simulink model "Nominal_CBF_ACC"  (R2018a)
settings: Solver=FixedStepAuto  StartTime=0.0  StopTime=Tsim  FixedStep=0.001  RelTol=1e-3
InitFcn:
  | tic;
  | disp('Simulation started...');
StopFcn:
  | elapsedTime_nominal = toc; % Stop timer when simulation ends
  | fprintf('Simulation Time: %.6f seconds\n', elapsedTime_nominal);
  | 
  | % out_nominal = out;
undefined symbols (not defined in the file): case_num, D0, epsilon, f0, f1, f2, g, gamma, k, k_fric, m, magnitude, omega0, p_omega, psc, v0, vd, x10, x20
settings Model: Creator=Administrator  LastModifiedBy=hieunguyen412
settings DataIOCC: ReturnWorkspaceOutputs=on
settings SFSimCC: SimUseLocalCustomCode=on
settings RTWCC: RTWUseLocalCustomCode=on

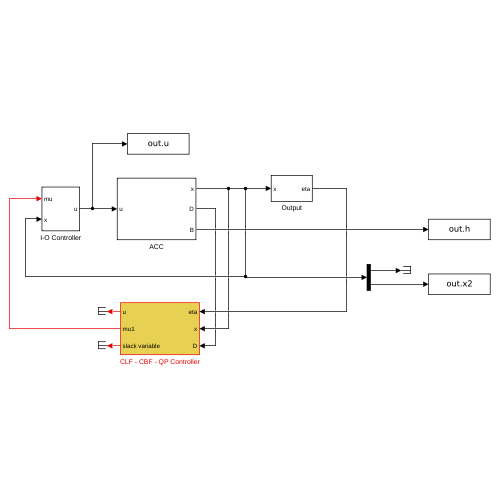
[thumbnail: Simulink's stored preview of the top-level diagram]
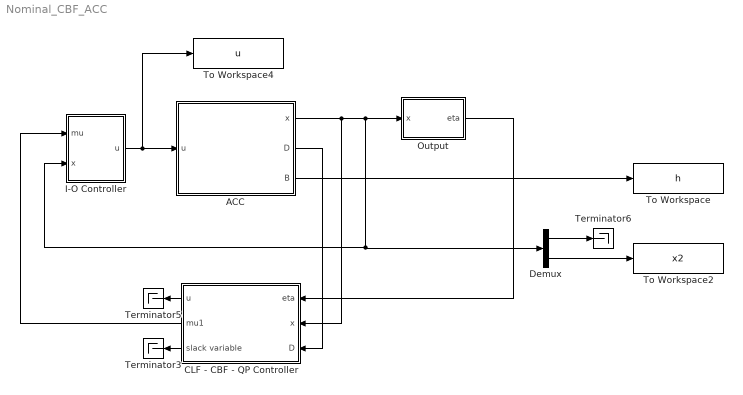
== system Nominal_CBF_ACC ==
  ACC : Subsystem
  CLF - CBF - QP Controller : Subsystem
  Demux : Demux  Outputs=2
  I-O Controller : Subsystem
  Output : Subsystem
  Terminator3 : Terminator
  Terminator5 : Terminator
  Terminator6 : Terminator
  To Workspace : ToWorkspace  VariableName=h  SampleTime=-1
  To Workspace2 : ToWorkspace  VariableName=x2  SampleTime=-1
  To Workspace4 : ToWorkspace  VariableName=u  SampleTime=-1
  wires:
  ACC/1(x) -> CLF - CBF - QP Controller/2(x), I-O Controller/2(x), Demux/1, Output/1(x)
  I-O Controller/1(u) -> To Workspace4/1, ACC/1(u)
  CLF - CBF - QP Controller/3(slack variable) -> Terminator3/1
  CLF - CBF - QP Controller/1(u) -> Terminator5/1
  ACC/2(D) -> CLF - CBF - QP Controller/3(D)
  Demux/1 -> Terminator6/1
  CLF - CBF - QP Controller/2(mu1) -> I-O Controller/1(mu)
  Demux/2 -> To Workspace2/1
  Output/1(eta) -> CLF - CBF - QP Controller/1(eta)
  ACC/3(B) -> To Workspace/1

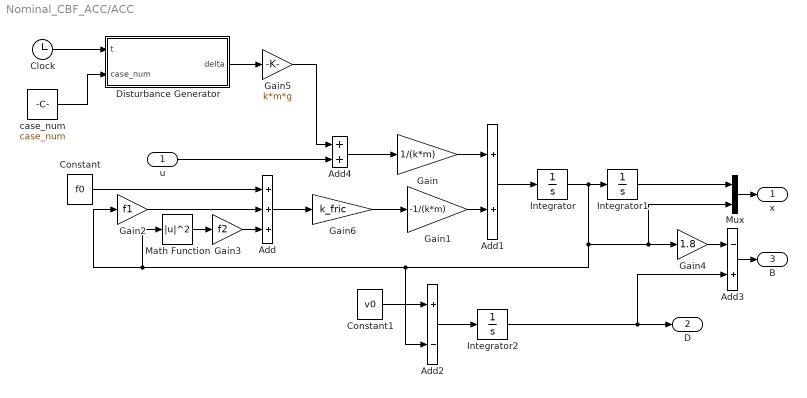
== system Nominal_CBF_ACC/ACC ==
  u : Inport  PortDimensions=1
  Add : Sum  Inputs=+++
  Add1 : Sum
  Add2 : Sum  Inputs=+-
  Add3 : Sum  Inputs=-+
  Add4 : Sum
  Clock : Clock
  Constant : Constant  Value=f0
  Constant1 : Constant  Value=v0
  Disturbance Generator : MATLAB Function  TreatAsAtomicUnit=on
  Gain : Gain  Gain=1/(k*m)
  Gain1 : Gain  Gain=-1/(k*m)
  Gain2 : Gain  Gain=f1
  Gain3 : Gain  Gain=f2
  Gain4 : Gain  Gain=1.8
  Gain5 : Gain  Gain=k*m*g
  Gain6 : Gain  Gain=k_fric
  Integrator : Integrator  InitialCondition=x20
  Integrator1 : Integrator  InitialCondition=x10
  Integrator2 : Integrator  InitialCondition=D0
  Math Function : Math  Operator=magnitude^2  SaturateOnIntegerOverflow=on
  Mux : Mux  Inputs=2
  case_num : Constant  Value=case_num
  x : Outport  PortDimensions=2
  D : Outport  Port=2  PortDimensions=1
  B : Outport  Port=3  PortDimensions=1
  wires:
  Constant/1 -> Add/1
  Gain2/1 -> Add/2
  Gain3/1 -> Add/3
  Gain/1 -> Add1/1
  Gain1/1 -> Add1/2
  Add1/1 -> Integrator/1
  Integrator/1 -> Add2/2, Math Function/1, Gain2/1, Mux/2, Gain4/1, Integrator1/1
  Math Function/1 -> Gain3/1
  Constant1/1 -> Add2/1
  Add2/1 -> Integrator2/1
  Integrator2/1 -> Add3/2, D/1
  Gain4/1 -> Add3/1
  Add3/1 -> B/1
  Mux/1 -> x/1
  Integrator1/1 -> Mux/1
  Disturbance Generator/1(delta) -> Gain5/1
  Clock/1 -> Disturbance Generator/1(t)
  Gain5/1 -> Add4/1
  Add4/1 -> Gain/1
  Add/1 -> Gain6/1
  Gain6/1 -> Gain1/1
  u/1 -> Add4/2
  case_num/1 -> Disturbance Generator/2(case_num)

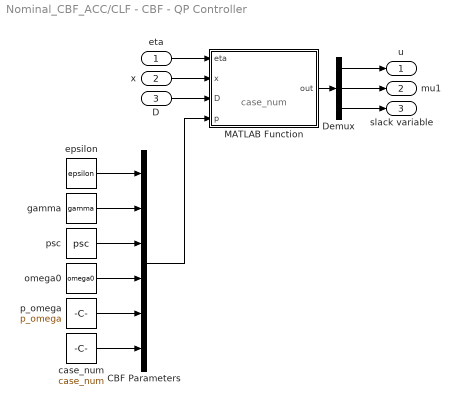
== system Nominal_CBF_ACC/CLF - CBF - QP Controller ==
  note: case_num
  eta : Inport  PortDimensions=1
  x : Inport  Port=2  PortDimensions=2
  D : Inport  Port=3  PortDimensions=1
  CBF Parameters : Mux  Inputs=6
  Demux : Demux  Outputs=3
  MATLAB Function : MATLAB Function  TreatAsAtomicUnit=on  SystemSampleTime=0.001
  case_num : Constant  Value=case_num
  epsilon : Constant  Value=epsilon
  gamma : Constant  Value=gamma
  omega0 : Constant  Value=omega0
  p_omega : Constant  Value=p_omega
  psc : Constant  Value=psc
  u : Outport  PortDimensions=1
  mu1 : Outport  Port=2  PortDimensions=1
  slack variable : Outport  Port=3  PortDimensions=1
  wires:
  Demux/3 -> slack variable/1
  eta/1 -> MATLAB Function/1(eta)
  D/1 -> MATLAB Function/3(D)
  Demux/2 -> mu1/1
  Demux/1 -> u/1
  x/1 -> MATLAB Function/2(x)
  MATLAB Function/1(out) -> Demux/1
  epsilon/1 -> CBF Parameters/1
  gamma/1 -> CBF Parameters/2
  CBF Parameters/1 -> MATLAB Function/4(p)
  psc/1 -> CBF Parameters/3
  omega0/1 -> CBF Parameters/4
  p_omega/1 -> CBF Parameters/5
  case_num/1 -> CBF Parameters/6

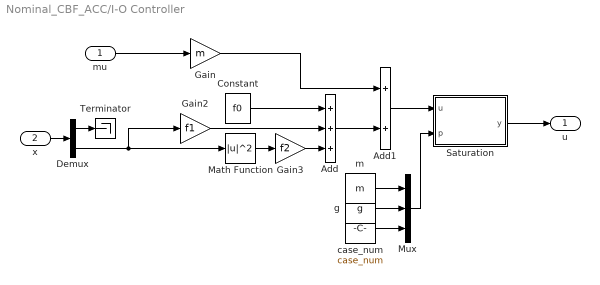
== system Nominal_CBF_ACC/I-O Controller ==
  mu : Inport
  x : Inport  Port=2  PortDimensions=2
  Add : Sum  Inputs=+++
  Add1 : Sum
  Constant : Constant  Value=f0
  Demux : Demux  Outputs=2
  Gain : Gain  Gain=m
  Gain2 : Gain  Gain=f1
  Gain3 : Gain  Gain=f2
  Math Function : Math  Operator=magnitude^2  SaturateOnIntegerOverflow=on
  Mux : Mux  Inputs=3
  Saturation : MATLAB Function  TreatAsAtomicUnit=on
  Terminator : Terminator
  case_num : Constant  Value=case_num
  g : Constant  Value=g
  m : Constant  Value=m
  u : Outport  PortDimensions=1
  wires:
  Gain3/1 -> Add/3
  Constant/1 -> Add/1
  Math Function/1 -> Gain3/1
  Gain2/1 -> Add/2
  Add/1 -> Add1/2
  mu/1 -> Gain/1
  Gain/1 -> Add1/1
  x/1 -> Demux/1
  Demux/2 -> Math Function/1, Gain2/1
  Demux/1 -> Terminator/1
  Add1/1 -> Saturation/1(u)
  Saturation/1(y) -> u/1
  case_num/1 -> Mux/3
  g/1 -> Mux/2
  m/1 -> Mux/1
  Mux/1 -> Saturation/2(p)

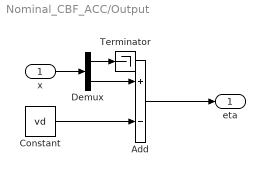
== system Nominal_CBF_ACC/Output ==
  x : Inport  PortDimensions=2
  Add : Sum  Inputs=+-
  Constant : Constant  Value=vd
  Demux : Demux  Outputs=2
  Terminator : Terminator
  eta : Outport  PortDimensions=1
  wires:
  Constant/1 -> Add/2
  Add/1 -> eta/1
  Demux/2 -> Add/1
  x/1 -> Demux/1
  Demux/1 -> Terminator/1

== matlab function Nominal_CBF_ACC/CLF - CBF - QP Controller/MATLAB Function ==
  data: eta input; out output; x input; D input; p input
function out = DO_QP_Controller(eta, x, D, p)
coder.extrinsic('quadprog');
out = zeros(3,1);

case_num = p(6);
if case_num == 1 || case_num == 2
    mode = 1;
else 
    mode = 2;
end
x2 = x(2); 

%% Physical parameters
m = 1650;
g = 9.81; 
f0 = 0.1;
f1 = 5;
f2 = 0.25;
vd = 24;
v0 =  13.89;

ca = 0.3;
cd = 0.3;

%% Controller parameters
epsilon = p(1); 
gamma = p(2);
psc = p(3);
omega0 = p(4); 
p_omega = p(5);

%% Aerodynamic drag force
Fr = f0 + f1*x2 + f2*x2.^2;

%% ============== QP 1 (No input saturation) ==============
if mode == 1
    %% CLF
    y = eta;
    V = y^2;
    LfV = 2*y*(-Fr/m); LgV = 2*y/m;
    A_clf = [LgV 0 -1]; b_clf = -LfV -epsilon*V;
    
    %% CBF
    B = D - 1.8*x2;
    LfB = v0 - x2 + 1.8*Fr/m;
    LgB = -1.8/m;
    A_cbf = [-LgB, 0, 0]; b_cbf = LfB + gamma*B;
    
    %% I-O L
    Lfy = -Fr/m; Lgy = 1/m;
    A_iol = [Lgy -1 0]; b_iol = - Lfy;
    
    %% QP
    A_ieq = [A_clf; A_cbf]; b_ieq = [b_clf; b_cbf];
    
    A_eq = A_iol; b_eq = b_iol;
    
    H_acc = [0, 0, 0; 0, 1, 0; 0, 0, psc];
    F_acc = [0; 0; 0];
    
    U = quadprog(H_acc, F_acc, A_ieq, b_ieq, A_eq, b_eq);
    
    out = U([1 2 3]);
end
%% ============== QP 2 (Optimal-decay variable included for handling input saturation) ==============
if mode == 2
    %============= CLF ============
    y = eta;
    V = y^2;
    LfV = 2*y*(-Fr/m); LgV = 2*y/m;
    A_clf = [LgV 0 -1 0]; b_clf = -LfV -epsilon*V;
    
    %============= CBF 1 ============
    h1 = D - 1.8*x2;
    Lfh1 = v0 - x2 + 1.8*Fr/m; Lgh1 = -1.8/m;
    A_cbf1 = [-Lgh1 0 0 -gamma*h1]; b_cbf1 = Lfh1 + omega0*gamma*h1;
    
    %============= I-O L ============
    Lfy = -Fr/m; Lgy = 1/m;
    A_iol = [Lgy -1 0 0]; b_iol = - Lfy;
    
    %============= Input constraints ============
    umax = ca*m*g; 
    umin = -cd*m*g;
    A_ic = [1 0 0 0; -1 0 0 0]; b_ic = [umax; -umin];
    
    %============= QP ============
    H_acc = [0, 0, 0, 0; 0, 1, 0, 0; 0, 0, psc, 0; 0, 0, 0, p_omega];
    F_acc = [0; 0; 0; 0];
    
    A_ieq = [A_clf; A_cbf1; A_ic]; b_ieq = [b_clf; b_cbf1; b_ic];
    
    A_eq = A_iol; b_eq = b_iol;
    
    U = quadprog(H_acc, F_acc, A_ieq, b_ieq, A_eq, b_eq);
    
    out = U([1 2 3]);
end

end

== matlab function Nominal_CBF_ACC/ACC/Disturbance Generator ==
  data: t input; delta output; case_num input
function delta = fcn(t, case_num)

if case_num == 1
    delta = 0.16*cos(2*pi*t/20) + 0.14*sin(2*pi*t/10 + pi/3);
elseif case_num == 2
    delta = 0.16*cos(2*pi*t/20) + 0.14*sin(2*pi*t/10 + pi/3);
else
    % delta = 0.18*cos(2*pi*t/20) + 0.14*sin(2*pi*t/10 - pi/8);
    delta = -(0.12*cos(2*pi*t/20) + 0.08*sin(2*pi*t/10 + pi/3));
end

== matlab function Nominal_CBF_ACC/I-O Controller/Saturation ==
  data: u input; y output; p input
function y = fcn(u, p)

m = p(1);
g = p(2);
case_num = p(3);

if case_num == 1 || case_num == 2
    y = u;
else
    if u >= 0.3*m*g
        y = 0.3*m*g;
    elseif u <= -0.3*m*g
        y = -0.3*m*g;
    else
        y = u;
    end
end

end
